simulink model "A2_suspension14"  (R2024a)
settings: Solver=ode45  StartTime=0.0  StopTime=10.0  FixedStep=0.001  MaxStep=0.01  RelTol=1e-3
values from neighbouring files (symbols this model uses):
  cs = data.cs    [A2_14.m]
  cw = (omega_n^2)*mw    [A2_14.m]
  ds = data.ds    [A2_14.m]
  dw = zeta*2*sqrt(cw*mw)    [A2_14.m]
  mc = data.mc    [A2_14.m]
  mw = data.mw    [A2_14.m]
settings Model: Creator=JonasMac  LastModifiedBy=testuser
settings SolverCC: AlgebraicLoopSolver=TrustRegion
settings DataIOCC: LimitDataPoints=on  SaveFormat=Array  SignalLoggingSaveFormat=ModelDataLogs  SaveTime=off  ReturnWorkspaceOutputs=off
settings OptimizationCC: BlockReduction=off  BooleanDataType=off  LifeSpan=inf
settings DebuggingCC: SaveWithParameterizedLinksMsg=none  UnderspecifiedInitializationDetection=Classic  MergeDetectMultiDrivingBlocksExec=none  SignalResolutionControl=TryResolveAllWithWarning  MultiTaskDSMMsg=warning  MultiTaskCondExecSysMsg=none  UnconnectedInputMsg=warning  UnconnectedOutputMsg=warning  UnconnectedLineMsg=warning  SFUnexpectedBacktrackingDiag=warning  SFNoUnconditionalDefaultTransitionDiag=warning  SFExecutionAtInitializationDiag=none  ArithmeticOperatorsInVariantConditions=warning
settings HardwareCC: ProdBitPerPointer=32  ProdBitPerSizeT=32  ProdBitPerPtrDiffT=32  ProdLargestAtomicFloat=None  ProdIntDivRoundTo=Undefined  ProdEndianess=Unspecified  ProdWordSize=32  ProdHWDeviceType=32-bit Generic  TargetUnknown=on
settings ModelReferenceCC: EnableRefExpFcnMdlSchedulingChecks=on  PropagateSignalLabelsOutOfModel=off
settings SFSimCC: SimUseLocalCustomCode=off  CustomCodeUndefinedFunction=UseInterfaceOnly
settings RTWCC: RTWUseLocalCustomCode=off  GPUComputeCapability=3.5  DLArmComputeVersion=19.05
settings CodeAppCC: StateflowObjectComments=on
settings GRTTargetCC: TargetLangStandard=C89/C90 (ANSI)
settings ConfigComp: CovMetricSettings=dw  CovSaveCumulativeToWorkspaceVar=on  CovSaveSingleToWorkspaceVar=on  CovExternalEMLEnable=off

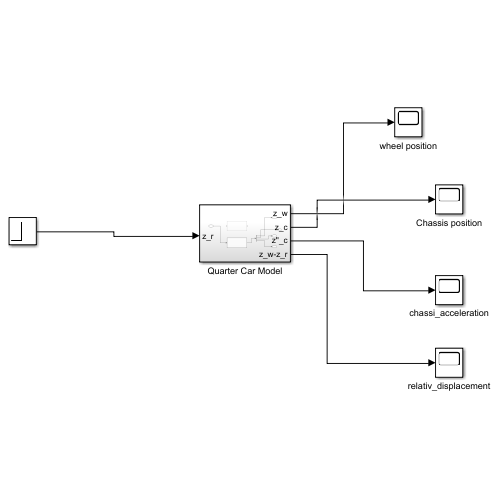
[thumbnail: Simulink's stored preview of the top-level diagram]
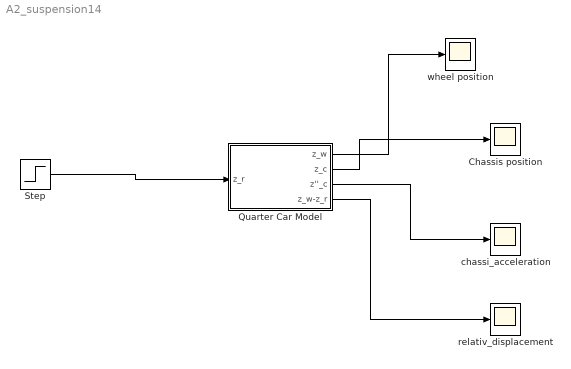
== system A2_suspension14 ==
  Chassis position : Scope
  Quarter Car Model : Subsystem
  Step : Step  After=0.05  SampleTime=0
  chassi_acceleration : Scope
  relativ_displacement : Scope
  wheel position : Scope
  wires:
  Quarter Car Model/2(z_c) -> Chassis position/1
  Step/1 -> Quarter Car Model/1(z_r)
  Quarter Car Model/1(z_w) -> wheel position/1
  Quarter Car Model/3(z''_c) -> chassi_acceleration/1
  Quarter Car Model/4(z_w-z_r) -> relativ_displacement/1

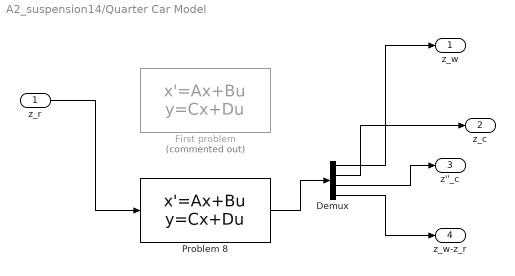
== system A2_suspension14/Quarter Car Model ==
  z_r : Inport
  Demux : Demux
  First problem : StateSpace  Commented=on  A=[0 1 0 0 ; -(cw+cs)/mw -(dw+ds)/mw (cs/mw) (ds/mw) ; 0 0 0 1 ; (cs/mc) (ds/mc) -(cs/mc) -(ds/mc)]  B=[0 ; cw/mw ; 0 ; 0]  C=[1 0 0 0 ; 0 0 1 0]  D=[0 ; 0]  InitialCondition=0
  Problem 8 : StateSpace  A=[0 1 0 0 ; -(cw+cs)/mw -(dw+ds)/mw (cs/mw) (ds/mw) ; 0 0 0 1 ; (cs/mc) (ds/mc) -(cs/mc) -(ds/mc)]  B=[0 ; cw/mw ; 0 ; 0]  C=[1 0 0 0; 0 0 1 0; cs/mc ds/mc -cs/mc -ds/mc; 1 0 0 0]  D=[0; 0; 0; -1]  InitialCondition=0
  z_w : Outport
  z_c : Outport  Port=2
  z''_c : Outport  Port=3
  z_w-z_r : Outport  Port=4
  wires:
  z_r/1 -> Problem 8/1
  Demux/1 -> z_w/1
  Demux/3 -> z''_c/1
  Demux/4 -> z_w-z_r/1
  Problem 8/1 -> Demux/1
  Demux/2 -> z_c/1
